simulink model "Logic_Calculator"  (R2016a)
settings: Solver=FixedStepDiscrete  StartTime=0.0  StopTime=10.0  RelTol=1e-3
libraries: simulink x6
settings Model: Creator=Muhammed  LastModifiedBy=Muhammed
settings OptimizationCC: DefaultParameterBehavior=Inlined  InlineInvariantSignals=on  EnableMemcpy=off  OptimizeModelRefInitCode=on  LifeSpan=1
settings DebuggingCC: UnderspecifiedInitializationDetection=Classic  MergeDetectMultiDrivingBlocksExec=none
settings ModelReferenceCC: PropagateSignalLabelsOutOfModel=off
settings RTWCC: SystemTargetFile=ert.tlc  GenCodeOnly=on  TemplateMakefile=ert_default_tmf  GenerateReport=on  IncludeHyperlinkInReport=on  LaunchReport=on  GenerateTraceInfo=on  GenerateTraceReport=on  GenerateTraceReportSl=on  GenerateTraceReportSf=on  GenerateTraceReportEml=on
settings CodeAppCC: ForceParamTrailComments=on  IgnoreCustomStorageClasses=off  OperatorAnnotations=on  SimulinkDataObjDesc=on  SFDataObjDesc=on  MATLABFcnDesc=on  InsertBlockDesc=on  MATLABSourceComments=on
settings ERTTargetCC: GenerateSampleERTMain=on  InlinedParameterPlacement=NonHierarchical  ERTCustomFileTemplate=example_file_process.tlc

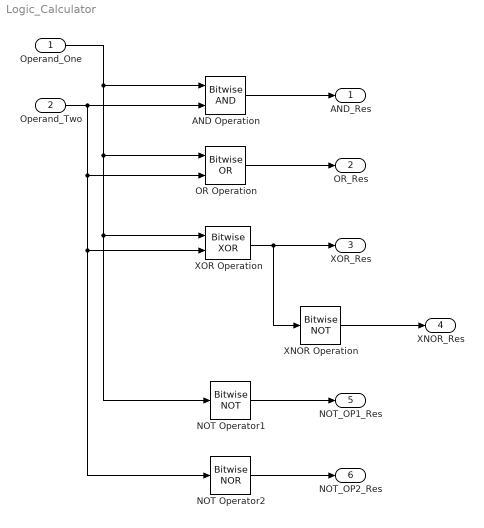
== system Logic_Calculator ==
  Operand_One : Inport  OutDataTypeStr=uint16
  Operand_Two : Inport  Port=2  OutDataTypeStr=uint16
  AND Operation : simulink/Logic and Bit Operations/Bitwise Operator  logicop=AND  UseBitMask=off  NumInputPorts=2  BitMask=bin2dec('11011001')  BitMaskRealWorld=Stored Integer
  NOT Operator1 : simulink/Logic and Bit Operations/Bitwise Operator  logicop=NOT  UseBitMask=off  BitMask=bin2dec('11011001')  BitMaskRealWorld=Stored Integer
  NOT Operator2 : simulink/Logic and Bit Operations/Bitwise Operator  logicop=NOR  UseBitMask=off  BitMask=bin2dec('11011001')  BitMaskRealWorld=Stored Integer
  OR Operation : simulink/Logic and Bit Operations/Bitwise Operator  logicop=OR  UseBitMask=off  NumInputPorts=2  BitMask=bin2dec('11011001')  BitMaskRealWorld=Stored Integer
  XNOR Operation : simulink/Logic and Bit Operations/Bitwise Operator  logicop=NOT  UseBitMask=off  BitMask=bin2dec('11011001')  BitMaskRealWorld=Stored Integer
  XOR Operation : simulink/Logic and Bit Operations/Bitwise Operator  logicop=XOR  UseBitMask=off  NumInputPorts=2  BitMask=bin2dec('11011001')  BitMaskRealWorld=Stored Integer
  AND_Res : Outport
  OR_Res : Outport  Port=2
  XOR_Res : Outport  Port=3
  XNOR_Res : Outport  Port=4
  NOT_OP1_Res : Outport  Port=5
  NOT_OP2_Res : Outport  Port=6
  wires:
  Operand_Two/1 -> XOR Operation/2, NOT Operator2/1, OR Operation/2, AND Operation/2
  OR Operation/1 -> OR_Res/1
  AND Operation/1 -> AND_Res/1
  Operand_One/1 -> AND Operation/1, NOT Operator1/1, XOR Operation/1, OR Operation/1
  NOT Operator1/1 -> NOT_OP1_Res/1
  NOT Operator2/1 -> NOT_OP2_Res/1
  XNOR Operation/1 -> XNOR_Res/1
  XOR Operation/1 -> XNOR Operation/1, XOR_Res/1
